simulink model "comparing21"  (R2021a)
settings: Solver=ode45  StartTime=0.0  StopTime=5  RelTol=1e-6  EnableMultiTasking=on
values from neighbouring files (symbols this model uses):
  sys = ss(A,B,C,D)    [linearization.m]
undefined symbols (not defined in the file or in its folder): x0_quadcopter
settings Model: Creator=Mauricio  LastModifiedBy=martijndebeuf
settings SolverCC: AlgebraicLoopSolver=TrustRegion
settings DataIOCC: LimitDataPoints=on  SaveFormat=Array  ReturnWorkspaceOutputs=off
settings OptimizationCC: ExpressionDepthLimit=2147483647  LifeSpan=inf
settings DebuggingCC: UnderspecifiedInitializationDetection=Classic  MergeDetectMultiDrivingBlocksExec=none  SolverPrmCheckMsg=warning  StateNameClashWarn=warning  SFUnexpectedBacktrackingDiag=warning  SFNoUnconditionalDefaultTransitionDiag=warning  SFExecutionAtInitializationDiag=none  SFMachineParentedDataDiag=warning  ArithmeticOperatorsInVariantConditions=warning
settings HardwareCC: ProdBitPerPointer=32  ProdBitPerSizeT=32  ProdBitPerPtrDiffT=32  ProdLargestAtomicFloat=None  ProdIntDivRoundTo=Undefined  ProdEndianess=Unspecified  ProdWordSize=32  ProdHWDeviceType=32-bit Generic
settings ModelReferenceCC: PropagateSignalLabelsOutOfModel=off
settings SFSimCC: SimUseLocalCustomCode=off  CustomCodeUndefinedFunction=UseInterfaceOnly
settings RTWCC: RTWUseLocalCustomCode=off
settings CodeAppCC: StateflowObjectComments=on
settings GRTTargetCC: TargetLangStandard=C89/C90 (ANSI)
settings ConfigComp: CovMetricSettings=dw  CovSaveCumulativeToWorkspaceVar=on  CovSaveSingleToWorkspaceVar=on  CovExternalEMLEnable=off

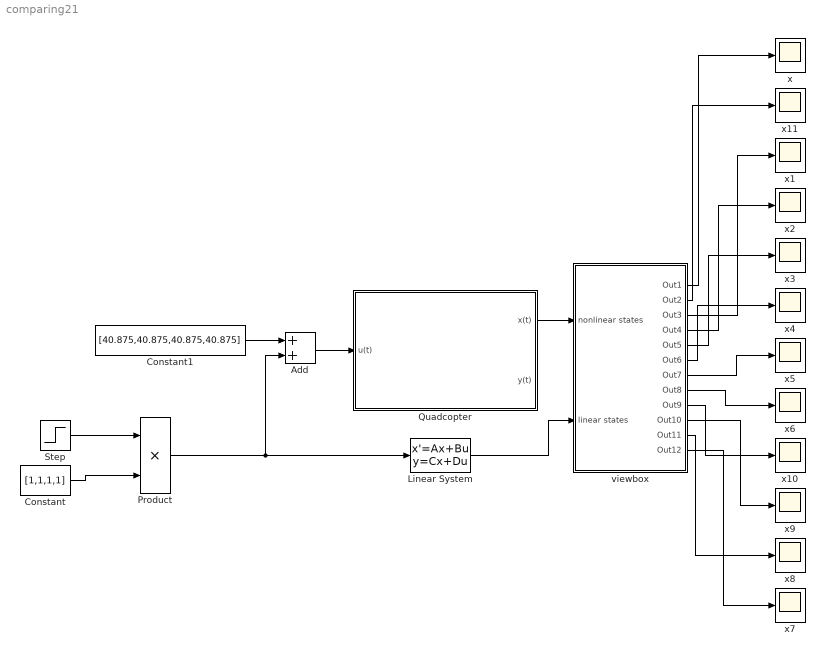
== system comparing21 ==
  Add : Sum
  Constant : Constant  Value=[1,1,1,1]
  Constant1 : Constant  Value=[40.875,40.875,40.875,40.875]
  "Linear System " : StateSpace  A=sys.A  B=sys.B  C=eye(12)  D=zeros(12,4)  InitialCondition=x0_quadcopter  ContinuousStateAttributes="\"states\""
  Product : Product
  Quadcopter : Subsystem  mask(Quadcopter){x0=x0_quadcopter, sel_payload=0}
      mask prompts: x0 "Initial State - x0:"; sel_payload "Payload [kg]:"
      mask help:
      | u(t): Vector containing the squared voltages of the motors
      |
      | Oscar Mauricio Agudelo
      | (c) 2013
      mask init:
      | switch sel_payload
      |     case 1
      |        payload=0; 
      |     case 2
      |        payload=0.1; 
      |     otherwise
      |         payload=0;
      | end
      mask TypeOptions sel_payload: 0 | 0.1
      mask Display:
      | image(imread('icon_quad.png'));
      | port_label('input',1,'u(t)')
      | port_label('output',1,'x(t)')
      | port_label('output',2,'y(t)')
  Step : Step  After=5  SampleTime=0
  viewbox : Subsystem
  x{,1..11} (12 alike) : Scope
  wires:
  Step/1 -> Product/1
  Constant/1 -> Product/2
  Constant1/1 -> Add/1
  Quadcopter/1(x(t)) -> viewbox/1(nonlinear states)
  "Linear System "/1 -> viewbox/2(linear states)
  viewbox/1(Out1) -> x/1
  Product/1 -> "Linear System "/1, Add/2
  Add/1 -> Quadcopter/1(u(t))
  viewbox/2(Out2) -> x11/1
  viewbox/3(Out3) -> x1/1
  viewbox/4(Out4) -> x2/1
  viewbox/5(Out5) -> x3/1
  viewbox/6(Out6) -> x4/1
  viewbox/7(Out7) -> x5/1
  viewbox/8(Out8) -> x6/1
  viewbox/9(Out9) -> x10/1
  viewbox/10(Out10) -> x9/1
  viewbox/11(Out11) -> x8/1
  viewbox/12(Out12) -> x7/1

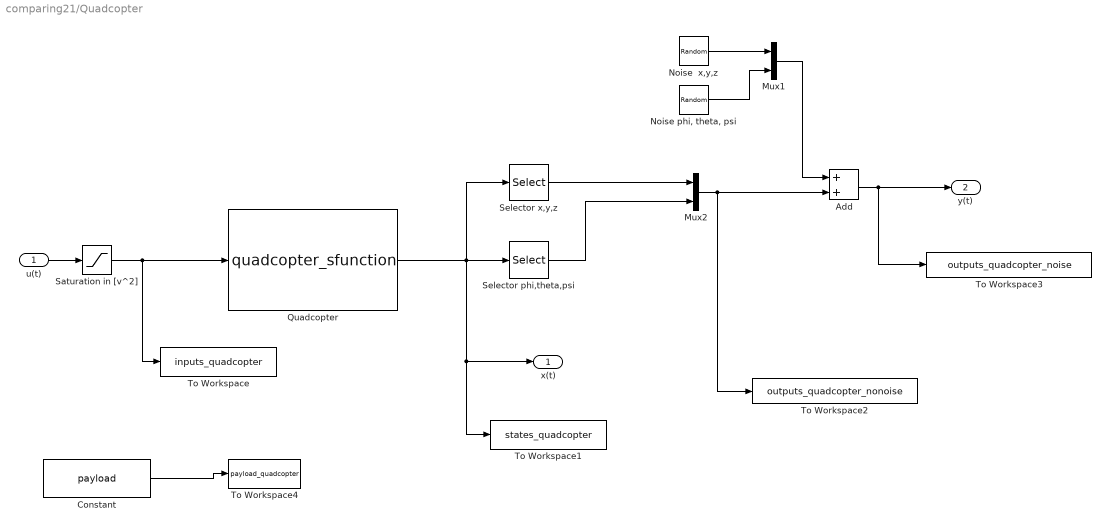
== system comparing21/Quadcopter ==
  u(t) : Inport
  Add : Sum
  Constant : Constant  Value=payload
  Mux1 : Mux  Inputs=2
  Mux2 : Mux  Inputs=2
  Noise  x,y,z : RandomNumber  Variance=[1 1 1]*(0.005)^2  SampleTime=0.05
  "Noise phi, theta, psi" : RandomNumber  Variance=[1 1 1]*(0.0087)^2  SampleTime=0.05
  Quadcopter : M-S-Function  FunctionName=quadcopter_sfunction  Parameters=x0, payload
  Saturation in [v^2] : Saturate  UpperLimit=100  LowerLimit=0
  Selector phi,theta,psi : Selector  IndexOptions=Index vector (dialog)  Indices=[7 8 9]  OutputSizes=1
  Selector x,y,z : Selector  IndexOptions=Index vector (dialog)  Indices=[1 2 3]  OutputSizes=1
  To Workspace : ToWorkspace  VariableName=inputs_quadcopter  SaveFormat=Structure With Time  SampleTime=-1
  To Workspace1 : ToWorkspace  VariableName=states_quadcopter  SaveFormat=Structure With Time  SampleTime=-1
  To Workspace2 : ToWorkspace  VariableName=outputs_quadcopter_nonoise  SaveFormat=Structure With Time  SampleTime=-1
  To Workspace3 : ToWorkspace  VariableName=outputs_quadcopter_noise  SaveFormat=Structure With Time  SampleTime=-1
  To Workspace4 : ToWorkspace  VariableName=payload_quadcopter  SampleTime=-1
  x(t) : Outport
  y(t) : Outport  Port=2
  wires:
  Saturation in [v^2]/1 -> Quadcopter/1, To Workspace/1
  u(t)/1 -> Saturation in [v^2]/1
  Mux2/1 -> To Workspace2/1, Add/2
  Selector phi,theta,psi/1 -> Mux2/2
  Selector x,y,z/1 -> Mux2/1
  Quadcopter/1 -> To Workspace1/1, x(t)/1, Selector x,y,z/1, Selector phi,theta,psi/1
  Add/1 -> To Workspace3/1, y(t)/1
  Noise  x,y,z/1 -> Mux1/1
  "Noise phi, theta, psi"/1 -> Mux1/2
  Mux1/1 -> Add/1
  Constant/1 -> To Workspace4/1

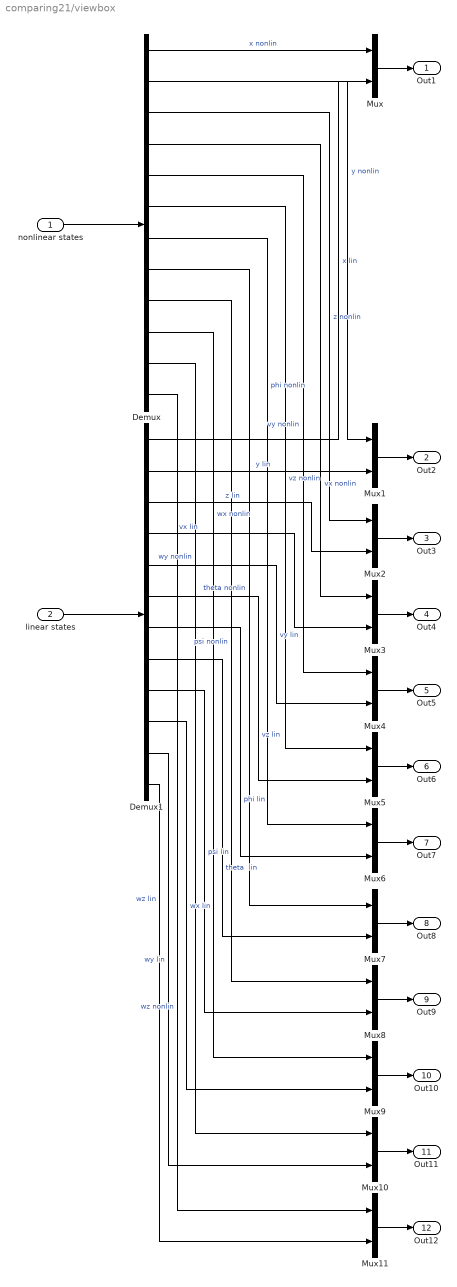
== system comparing21/viewbox ==
  nonlinear states : Inport
  linear states : Inport  Port=2
  Demux : Demux  Outputs=12
  Demux1 : Demux  Outputs=12
  Mux{,1..11} (12 alike) : Mux  Inputs=2
  Out1 : Outport
  Out2 : Outport  Port=2
  Out3 : Outport  Port=3
  Out4 : Outport  Port=4
  Out5 : Outport  Port=5
  Out6 : Outport  Port=6
  Out7 : Outport  Port=7
  Out8 : Outport  Port=8
  Out9 : Outport  Port=9
  Out10 : Outport  Port=10
  Out11 : Outport  Port=11
  Out12 : Outport  Port=12
  wires:
  Mux10/1 -> Out11/1
  Mux8/1 -> Out9/1
  Mux3/1 -> Out4/1
  Mux9/1 -> Out10/1
  Demux1/8 -> Mux7/2  "theta  lin"
  Demux1/1 -> Mux/2  "x lin"
  Demux/12 -> Mux11/1  "wz nonlin"
  Demux1/2 -> Mux1/2  "y lin"
  Demux1/9 -> Mux8/2  "psi lin"
  Mux1/1 -> Out2/1
  Demux1/3 -> Mux2/2  "z lin"
  Demux1/10 -> Mux9/2  "wx lin"
  Demux/3 -> Mux2/1  "z nonlin"
  Mux5/1 -> Out6/1
  Demux/4 -> Mux3/1  "vx nonlin"
  Demux1/5 -> Mux4/2  "vy lin"
  Demux1/11 -> Mux10/2  "wy lin"
  Mux4/1 -> Out5/1
  Demux/10 -> Mux9/1  "wx nonlin"
  Demux/1 -> Mux/1  "x nonlin"
  Demux/5 -> Mux4/1  "vy nonlin"
  Demux1/12 -> Mux11/2  "wz lin"
  Demux/6 -> Mux5/1  "vz nonlin"
  Demux/11 -> Mux10/1  "wy nonlin"
  Demux/7 -> Mux6/1  "phi nonlin"
  Mux6/1 -> Out7/1
  Mux/1 -> Out1/1
  Demux/9 -> Mux8/1  "psi nonlin"
  Demux1/4 -> Mux3/2  "vx lin"
  Mux2/1 -> Out3/1
  Demux/2 -> Mux1/1  "y nonlin"
  Demux/8 -> Mux7/1  "theta nonlin"
  linear states/1 -> Demux1/1
  Demux1/7 -> Mux6/2  "phi lin"
  Mux11/1 -> Out12/1
  Demux1/6 -> Mux5/2  "vz lin"
  Mux7/1 -> Out8/1
  nonlinear states/1 -> Demux/1
